simulink model "modelloSatelliteControlloAdattativo"  (R2025b)
settings: Solver=ode45  StartTime=0.0  StopTime=50  MaxStep=1e-3  RelTol=1e-3
values from neighbouring files (symbols this model uses):
  I = [13470; 20450; 27200]    [main.m]
  K = diag([4 4 4])    [main.m]
  rho = [30; 30; 30]    [main.m]
settings Model: Creator=Armando  LastModifiedBy=Armando

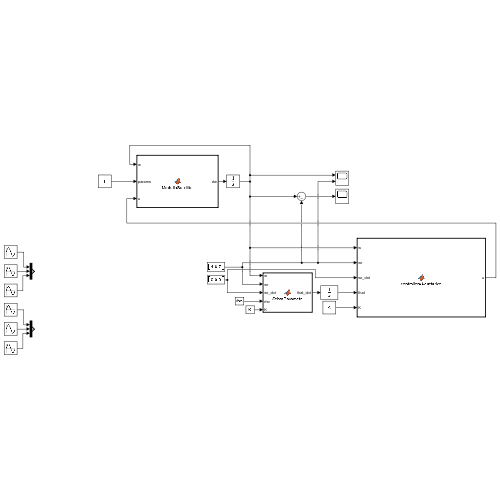
[thumbnail: Simulink's stored preview of the top-level diagram]
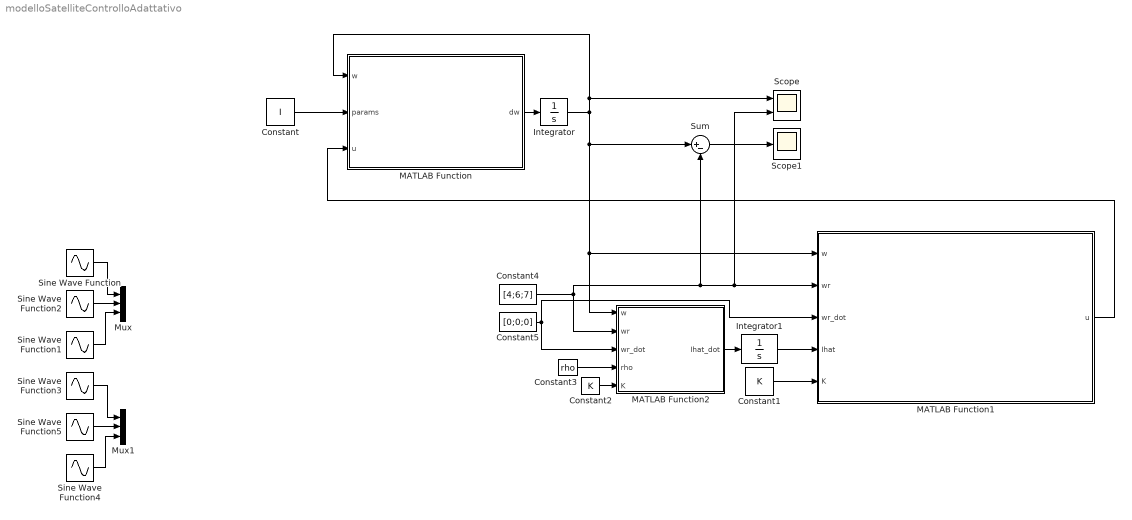
== system modelloSatelliteControlloAdattativo ==
  Constant : Constant  Value=I
  Constant1 : Constant  Value=K
  Constant2 : Constant  Value=K
  Constant3 : Constant  Value=rho
  Constant4 : Constant  Value=[4;6;7]
  Constant5 : Constant  Value=[0;0;0]
  Integrator : Integrator  InitialCondition=[1;1;-1]
  Integrator1 : Integrator  InitialCondition=[1;1;1]
  MATLAB Function : MATLAB Function  TreatAsAtomicUnit=on
  MATLAB Function1 : MATLAB Function  TreatAsAtomicUnit=on
  MATLAB Function2 : MATLAB Function  TreatAsAtomicUnit=on
  Mux : Mux  Inputs=3
  Mux1 : Mux  Inputs=3
  Scope : Scope  NumInputPorts=2
      settings: ActiveDisplayYMinimum=-1.3137144511748584  ActiveDisplayYMaximum=9.2277728766856963
  Scope1 : Scope
      settings: ActiveDisplayYMinimum=-9.3981952442908234  ActiveDisplayYMaximum=4.5484867263666384
  Sine Wave Function : Sin  SampleTime=0
  Sine Wave Function1 : Sin  Amplitude=2  SampleTime=0
  Sine Wave Function2 : Sin  Amplitude=4  SampleTime=0
  Sine Wave Function3 : Sin  Frequency=0  Phase=pi/2  SampleTime=0
  Sine Wave Function4 : Sin  Amplitude=2  Phase=pi/2  SampleTime=0
  Sine Wave Function5 : Sin  Amplitude=4  Phase=pi/2  SampleTime=0
  Sum : Sum  Inputs=|+-
  wires:
  Constant/1 -> MATLAB Function/2(params)
  MATLAB Function/1(dw) -> Integrator/1
  Integrator/1 -> Sum/1, MATLAB Function2/1(w), MATLAB Function1/1(w), Scope/1, MATLAB Function/1(w)
  Constant1/1 -> MATLAB Function1/5(K)
  Sine Wave Function/1 -> Mux/1
  Sine Wave Function2/1 -> Mux/2
  Sine Wave Function1/1 -> Mux/3
  Constant2/1 -> MATLAB Function2/5(K)
  Constant3/1 -> MATLAB Function2/4(rho)
  MATLAB Function1/1(u) -> MATLAB Function/3(u)
  Integrator1/1 -> MATLAB Function1/4(Ihat)
  Sine Wave Function5/1 -> Mux1/2
  Sine Wave Function4/1 -> Mux1/3
  Sine Wave Function3/1 -> Mux1/1
  Sum/1 -> Scope1/1
  MATLAB Function2/1(Ihat_dot) -> Integrator1/1
  Constant4/1 -> MATLAB Function2/2(wr), Sum/2, Scope/2, MATLAB Function1/2(wr)
  Constant5/1 -> MATLAB Function2/3(wr_dot), MATLAB Function1/3(wr_dot)

== matlab function modelloSatelliteControlloAdattativo/MATLAB Function1 ==
  data: w input; u output; wr input; wr_dot input; Ihat input; K input
function u = controlloreAdattativo(w, wr, wr_dot, Ihat, K)

    I1 = Ihat(1);I2 = Ihat(2);I3 = Ihat(3);

   
    e = w - wr;
    k1 = K(1,1);k2 = K(2,2);k3 = K(3,3);

    u1 = I1*(wr_dot(1) - k1*e(1)) - (I2-I3)*w(2)*w(3);
    u2 = I2*(wr_dot(2) - k2*e(2)) - (I3-I1)*w(1)*w(3);
    u3 = I3*(wr_dot(3) - k3*e(3)) - (I1-I2)*w(1)*w(2);

    u = [u1; u2; u3];
end

== matlab function modelloSatelliteControlloAdattativo/MATLAB Function ==
  data: w input; dw output; params input; u input
function dw = ModelloSatellite(w,params,u)
    c = [(params(2) - params(3))/params(1)*w(2)*w(3);
         ( params(3)- params(1))/params(2)*w(3)*w(1);
          (params(1) - params(2))/params(3)*w(1)*w(2)];
    
    dw = c + (u./params(:));

== matlab function modelloSatelliteControlloAdattativo/MATLAB Function2 ==
  data: w input; Ihat_dot output; wr input; wr_dot input; rho input; K input
function Ihat_dot = StimaParametri(w, wr, wr_dot, rho, K)

    % Errori di tracking
    e = w - wr;

    % Guadagni
    k1 = K(1,1);k2 = K(2,2);k3 = K(3,3);     
    
    Ihat_dot_1 = rho(1) * (e(1)*(k1*e(1) - wr_dot(1)) - e(2)*w(1)*w(3) + e(3)*w(1)*w(2) );
    Ihat_dot_2 = rho(2) * (e(2)*(k2*e(2) - wr_dot(2)) + e(1)*w(2)*w(3) - e(3)*w(1)*w(2) );
    Ihat_dot_3 = rho(3) * (e(3)*(k3*e(3) - wr_dot(3)) - e(1)*w(2)*w(3) + e(2)*w(1)*w(3) );


    Ihat_dot = [Ihat_dot_1; Ihat_dot_2;Ihat_dot_3];

end
